simulink model "lqrModel"  (R2020b)
settings: Solver=VariableStepAuto  StartTime=0.0  StopTime=10.0  RelTol=1e-3
InitFcn:
  | lqrDesign
undefined symbols (not defined in the file or in its folder): K
settings Model: Creator=kuzub  LastModifiedBy=kuzub

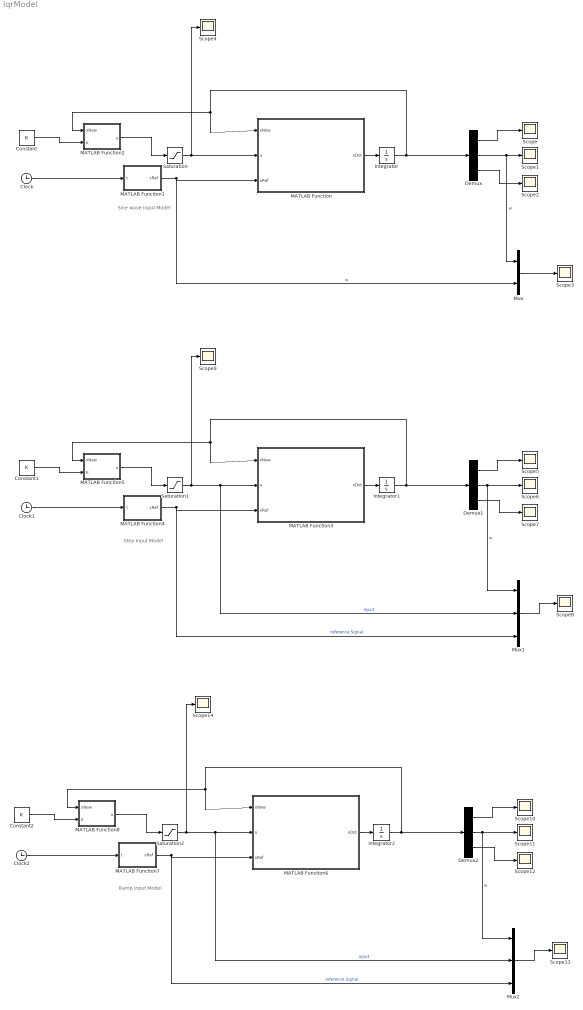
== system lqrModel ==
  note: Step Input Model
  note: Sine wave Input Model
  note: Ramp Input Model
  Clock : Clock
  Clock1 : Clock
  Clock2 : Clock
  Constant : Constant  Value=K  VectorParams1D=off
  Constant1 : Constant  Value=K  VectorParams1D=off
  Constant2 : Constant  Value=K  VectorParams1D=off
  Demux : Demux  Outputs=3
  Demux1 : Demux  Outputs=3
  Demux2 : Demux  Outputs=3
  Integrator : Integrator  InitialCondition=[0;0;0]
  Integrator1 : Integrator  InitialCondition=[0;0;0]
  Integrator2 : Integrator  InitialCondition=[0;0;0]
  MATLAB Function : MATLAB Function  TreatAsAtomicUnit=on
  MATLAB Function1 : MATLAB Function  TreatAsAtomicUnit=on
  MATLAB Function2 : MATLAB Function  TreatAsAtomicUnit=on
  MATLAB Function3 : MATLAB Function  TreatAsAtomicUnit=on
  MATLAB Function4 : MATLAB Function  TreatAsAtomicUnit=on
  MATLAB Function5 : MATLAB Function  TreatAsAtomicUnit=on
  MATLAB Function6 : MATLAB Function  TreatAsAtomicUnit=on
  MATLAB Function7 : MATLAB Function  TreatAsAtomicUnit=on
  MATLAB Function8 : MATLAB Function  TreatAsAtomicUnit=on
  Mux : Mux  Inputs=2
  Mux1 : Mux  Inputs=3
  Mux2 : Mux  Inputs=3
  Saturation : Saturate  UpperLimit=20  LowerLimit=0
  Saturation1 : Saturate  UpperLimit=20  LowerLimit=0
  Saturation2 : Saturate  UpperLimit=20  LowerLimit=0
  Scope{,1..14} (15 alike) : Scope
  wires:
  MATLAB Function/1(xDot) -> Integrator/1
  Integrator/1 -> Demux/1, MATLAB Function/1(xNew), MATLAB Function2/1(xNew)
  Clock/1 -> MATLAB Function1/1(t)
  MATLAB Function2/1(u) -> Saturation/1
  MATLAB Function1/1(xRef) -> Mux/2, MATLAB Function/3(xRef)  "w"
  Constant/1 -> MATLAB Function2/2(K)
  Demux/1 -> Scope/1
  Demux/2 -> Mux/1, Scope1/1  "w"
  Demux/3 -> Scope2/1
  Mux/1 -> Scope3/1
  Saturation/1 -> MATLAB Function/2(u), Scope4/1
  Saturation1/1 -> Scope9/1, Mux1/2, MATLAB Function3/2(u)  "input"
  Mux1/1 -> Scope8/1
  Demux1/3 -> Scope7/1
  Demux1/2 -> Scope6/1, Mux1/1  "w"
  Demux1/1 -> Scope5/1
  Constant1/1 -> MATLAB Function5/2(K)
  MATLAB Function4/1(xRef) -> MATLAB Function3/3(xRef), Mux1/3  "reference Signal"
  MATLAB Function5/1(u) -> Saturation1/1
  Clock1/1 -> MATLAB Function4/1(t)
  Integrator1/1 -> MATLAB Function5/1(xNew), MATLAB Function3/1(xNew), Demux1/1
  MATLAB Function3/1(xDot) -> Integrator1/1
  MATLAB Function6/1(xDot) -> Integrator2/1
  Integrator2/1 -> Demux2/1, MATLAB Function6/1(xNew), MATLAB Function8/1(xNew)
  Clock2/1 -> MATLAB Function7/1(t)
  MATLAB Function8/1(u) -> Saturation2/1
  MATLAB Function7/1(xRef) -> Mux2/3, MATLAB Function6/3(xRef)  "reference Signal"
  Constant2/1 -> MATLAB Function8/2(K)
  Demux2/1 -> Scope10/1
  Demux2/2 -> Mux2/1, Scope11/1  "w"
  Demux2/3 -> Scope12/1
  Mux2/1 -> Scope13/1
  Saturation2/1 -> MATLAB Function6/2(u), Mux2/2, Scope14/1  "input"

== matlab function lqrModel/MATLAB Function ==
  data: xNew input; u input; xDot output; xRef input
function xDot = fcn(xNew, u, xRef)
    %
    %%% System Constants
    R = 0.55;
    J = 0.09;
    Kt = 85*10^-3;
    L = 25*10^-3;
    b = 0.05;
    %
    %%% State Space Matrix
    %
    a00 = -R/L;
    a01 = -Kt/L;
    a10 = Kt/J;
    a11 = -b/J;
    %
    b00 = 1/L;
    b10 = 0;
    %
    A = [a00, a01;
         a10, a11];
    % 
    B = [b00; b10];
    
    %%% Reference Tracking 
    Anew = [A, zeros(2,1);
            0, 1, 0];
    %
    Bnew = [B;
            0];
    %
    eRef = [0; 
            0; 
            -1];
    %
    xDot = Anew*xNew + Bnew*u + eRef*xRef;
end

== matlab function lqrModel/MATLAB Function2 ==
  data: xNew input; u output; K input
function u = fcn(xNew, K)



u = -K*xNew; 
end

== matlab function lqrModel/MATLAB Function3 ==
  data: xNew input; u input; xDot output; xRef input
function xDot = fcn(xNew, u, xRef)
    %
    %%% System Constants
    R = 0.55;
    J = 0.09;
    Kt = 85*10^-3;
    L = 25*10^-3;
    b = 0.05;
    %
    %%% State Space Matrix
    %
    a00 = -R/L;
    a01 = -Kt/L;
    a10 = Kt/J;
    a11 = -b/J;
    %
    b00 = 1/L;
    b10 = 0;
    %
    A = [a00, a01;
         a10, a11];
    % 
    B = [b00; b10];
    
    %%% Reference Tracking 
    Anew = [A, zeros(2,1);
            0, 1, 0];
    %
    Bnew = [B;
            0];
    %
    eRef = [0; 
            0; 
            -1];
    %
    xDot = Anew*xNew + Bnew*u + eRef*xRef;
end

== matlab function lqrModel/MATLAB Function4 ==
  data: t input; xRef output
function xRef = fcn(t)
    %
    f = 0.1;
    %
    A = 5;
    %A = 0;
    %
    bias = 10;
    %
    %xRef = bias + A*sin(2*pi*f*t);
    xRef = bias;
end

== matlab function lqrModel/MATLAB Function5 ==
  data: xNew input; u output; K input
function u = fcn(xNew, K)



u = -K*xNew; 
end

== matlab function lqrModel/MATLAB Function6 ==
  data: xNew input; u input; xDot output; xRef input
function xDot = fcn(xNew, u, xRef)
    %
    %%% System Constants
    R = 0.55;
    J = 0.09;
    Kt = 85*10^-3;
    L = 25*10^-3;
    b = 0.05;
    %
    %%% State Space Matrix
    %
    a00 = -R/L;
    a01 = -Kt/L;
    a10 = Kt/J;
    a11 = -b/J;
    %
    b00 = 1/L;
    b10 = 0;
    %
    A = [a00, a01;
         a10, a11];
    % 
    B = [b00; b10];
    
    %%% Reference Tracking 
    Anew = [A, zeros(2,1);
            0, 1, 0];
    %
    Bnew = [B;
            0];
    %
    eRef = [0; 
            0; 
            -1];
    %
    xDot = Anew*xNew + Bnew*u + eRef*xRef;
end

== matlab function lqrModel/MATLAB Function7 ==
  data: t input; xRef output
function xRef = fcn(t)
    %
    f = 0.1;
    %
    A = 5;
    %A = 0;
    %
    bias = 10;
    %
    %xRef = bias + A*sin(2*pi*f*t);
    xRef = bias;
end

== matlab function lqrModel/MATLAB Function8 ==
  data: xNew input; u output; K input
function u = fcn(xNew, K)



u = -K*xNew; 
end

== matlab function lqrModel/MATLAB Function1 ==
  data: t input; xRef output
function xRef = fcn(t)
    %
    f = 0.1;
    %
    A = 5;
    %A = 0;
    %
    bias = 10;
    %
    xRef = bias + A*sin(2*pi*f*t);
end
